simulink model "gain_scheduling_controlloreP"  (R2023b)
settings: Solver=VariableStepAuto  StartTime=0.0  StopTime=20  RelTol=1e-3
values from neighbouring files (symbols this model uses):
  A_lin = double(A_lin)    [WP5.m]
  B_lin = double(B_lin)    [WP5.m]
  C_lin = [1 0]    [WP5.m]
  D_lin = 0    [WP5.m]
  Kp_sigma = double(subs(kp.kp, 'sigma', r))    [WP5.m]
  r = 0.0451    [WP5.m]
  x1_eq = double(x1_eq)    [WP5.m]    (also in WP5_lqr.m = sol.x1(1); prova_GS_sf_IA.m = sol.x1)
  x2_eq = double(x2_eq)    [WP5.m]    (also in WP5_lqr.m = sol.x2(1); prova_GS_sf_IA.m = sol.x2)
settings Model: Creator=kiraa  LastModifiedBy=kiraa

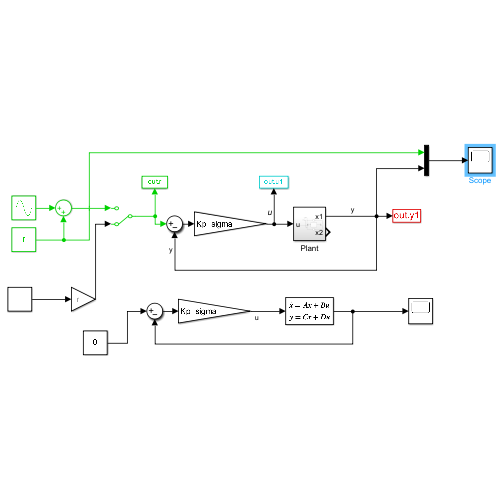
[thumbnail: Simulink's stored preview of the top-level diagram]
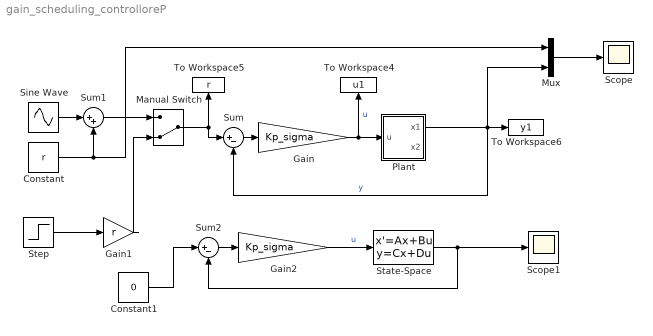
== system gain_scheduling_controlloreP ==
  Constant : Constant  Value=r
  Constant1 : Constant  Value=0
  Gain : Gain  Gain=Kp_sigma
  Gain1 : Gain  Gain=r
  Gain2 : Gain  Gain=Kp_sigma
  Manual Switch : ManualSwitch  CurrentSetting=0
  Mux : Mux  Inputs=2
  Plant : Subsystem
  Scope : Scope
  Scope1 : Scope
  Sine Wave : Sin  Amplitude=0.5  Frequency=0.5  SampleTime=0
  State-Space : StateSpace  A=A_lin  B=B_lin  C=C_lin  D=D_lin  InitialCondition=[1 1]
  Step : Step  Time=3  SampleTime=0
  Sum : Sum  Inputs=|+-
  Sum1 : Sum  Inputs=|++
  Sum2 : Sum  Inputs=|+-
  To Workspace4 : ToWorkspace  VariableName=u1  SaveFormat=Timeseries  SampleTime=-1
  To Workspace5 : ToWorkspace  VariableName=r  SaveFormat=Timeseries  SampleTime=-1
  To Workspace6 : ToWorkspace  VariableName=y1  SaveFormat=Timeseries  SampleTime=-1
  wires:
  Constant/1 -> Sum1/2, Mux/1
  Sine Wave/1 -> Sum1/1
  Gain/1 -> Plant/1(u), To Workspace4/1  "u"
  Sum/1 -> Gain/1
  Sum1/1 -> Manual Switch/1
  Plant/1(x1) -> Mux/2, Sum/2, To Workspace6/1  "y"
  Manual Switch/1 -> Sum/1, To Workspace5/1
  Mux/1 -> Scope/1
  Step/1 -> Gain1/1
  Gain1/1 -> Manual Switch/2
  Gain2/1 -> State-Space/1  "u"
  Sum2/1 -> Gain2/1
  State-Space/1 -> Scope1/1, Sum2/2
  Constant1/1 -> Sum2/1

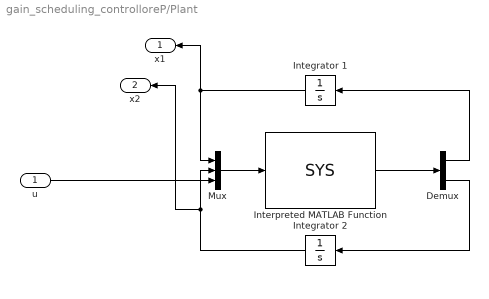
== system gain_scheduling_controlloreP/Plant ==
  u : Inport
  Demux : Demux  Outputs=2
  Integrator 1 : Integrator  InitialCondition=x1_eq
  Integrator 2 : Integrator  InitialCondition=x2_eq
  Interpreted MATLAB Function : MATLABFcn  MATLABFcn=SYS  OutputDimensions=2
  Mux : Mux  Inputs=3
  x1 : Outport
  x2 : Outport  Port=2
  wires:
  u/1 -> Mux/3
  Demux/2 -> Integrator 2/1
  Interpreted MATLAB Function/1 -> Demux/1
  Integrator 2/1 -> Mux/2, x2/1
  Mux/1 -> Interpreted MATLAB Function/1
  Demux/1 -> Integrator 1/1
  Integrator 1/1 -> Mux/1, x1/1
